simulink library "PB_Library_Master_Working"  (R2021a)
settings: Solver=VariableStepAuto  StartTime=0.0  StopTime=10.0  RelTol=1e-3
undefined symbols (not defined in the file): A_M, B_M, component_degradation_input, E0_M, f_sw, f_sw_M_aDF, flux_m_aDF, Fsw_M_aDF, insert, K_M, L_M_aDF, L_M_adf, P_Fe_Nom_aDF, Q_M, Q_rr, r_c, r_D, R_M, R_s_aDF, resistance_aDF, S_nom_aDF, SOC_Init_M, TFall_M_aDF, TRise_M_aDF, Trr_M_aDF, u_ce0, u_D0
libraries: $bdroot x76, Lib_Dyn_StateSpace_EMTAT x6, Lib_PF_BusLoadDC_TMATS x3, PB_Library_Master x3, simulink x3, TemperatureBlock x1
(part 2 of 5)

== system PB_Library_Master_Working/Boost Converter ==
  Vin : Inport
  IgIn : Inport  Port=2
  x : Inport  Port=3
  d : Inport  Port=4
  dt : Inport  Port=5
  Iout : Inport  Port=6
  Temp (Rankine) : Inport  Port=7  Unit=degC
  Bus : Lib_PF_BusLoadDC_TMATS/LoadBus DC  P_M=-Pdis_M  BlkNm_M=double(gcb)
  Bus Creator : BusCreator  Inputs=11
  DC - DC Converter : Subsystem
      mask Display:
      | fprintf('Boost')
      | 
      | port_label('input',1,'VA')
      | port_label('input',2,'IAg')
      | port_label('input',3,'x')
      | port_label('input',4,'d')
      | port_label('input',5,'dt')
      | port_label('input',6,'Iout')
      | port_label('input',7,'Ploss')
      | 
      | 
      | port_label('output',1,'VB')
      | port_label('output',2,'x_dot')
      | port_label('output',3,'x_new')
      | port_label('output',4,'PElec')
      | port_label('output',5,'IA')
      | port_label('output',6,'switchDyn')
  Display : Display
  "Power Loss " : Subsystem
  Product1 : Product
  Product3 : Product
  Rankine to Celsius : PB_Library_Master/Rankine to Celsius  SystemSampleTime=-1  VariantActivationTime=update diagram  Latency=0  AutoFrameSizeCalculation=off
  "TempConv " : Subsystem  Commented=on
      mask DialogControl DescTextVar Prompt: Temperature Unit Converter
  Terminator3 : Terminator
  Vout : Outport  VectorParamsAs1DForOutWhenUnconnected=off
  xdot : Outport  Port=2  VectorParamsAs1DForOutWhenUnconnected=off
  x_new : Outport  Port=3  VectorParamsAs1DForOutWhenUnconnected=off
  P_err : Outport  Port=4  VectorParamsAs1DForOutWhenUnconnected=off
  Outputs : Outport  Port=5  VectorParamsAs1DForOutWhenUnconnected=off
  Iin : Outport  Port=6  VectorParamsAs1DForOutWhenUnconnected=off
  Heat (W) : Outport  Port=7  VectorParamsAs1DForOutWhenUnconnected=off
  wires:
  DC - DC Converter/4(PElec) -> Bus/2
  Temp (Rankine)/1 -> Rankine to Celsius/1, Display/1  "TempIn"
  Rankine to Celsius/1 -> DC - DC Converter/8("T_Ambient "), "Power Loss "/5("T_Ambient ")
  DC - DC Converter/6(switchDyn) -> Bus Creator/1  "switchDyn"
  dt/1 -> DC - DC Converter/5(dt)
  DC - DC Converter/3(x_new) -> x_new/1, Bus Creator/10  "x"
  "Power Loss "/1(" P loss") -> Heat (W)/1, Bus Creator/3, DC - DC Converter/7(P loss)  "P loss"
  d/1 -> DC - DC Converter/4(d), "Power Loss "/3(d)
  x/1 -> DC - DC Converter/3(x)
  IgIn/1 -> DC - DC Converter/2(IAg)
  DC - DC Converter/5(IA) -> Iin/1, Bus Creator/2, Product3/2  "Iin"
  DC - DC Converter/2(x_dot) -> xdot/1, Bus Creator/11  "x_dot"
  Iout/1 -> Bus Creator/5, Product1/1, Bus/3, "Power Loss "/2(Iout), DC - DC Converter/6(Iout)  "Iout"
  Bus/1 -> Vout/1, "Power Loss "/4(Vout)
  Product1/1 -> Bus Creator/7  "Pout"
  Product3/1 -> Bus Creator/6  "Pin"
  Vin/1 -> Bus Creator/4, Product3/1, "Power Loss "/1(Vin), DC - DC Converter/1(NodeA)  "Vin"
  DC - DC Converter/1(NodeB) -> Bus/1, Product1/2
  Bus/3 -> Terminator3/1
  Bus/2 -> P_err/1
  Bus Creator/1 -> Outputs/1
  "Power Loss "/3(RippleV) -> Bus Creator/9  "Ripple V"
  "Power Loss "/2(RippleI) -> Bus Creator/8  "Ripple I"

== system PB_Library_Master_Working/Boost Converter Analytic ==
  Vin : Inport
  x : Inport  Port=2
  d : Inport  Port=3
  dt : Inport  Port=4
  Iout : Inport  Port=5
  Temp (Rankine) : Inport  Port=6  Unit=degC
  FaultToggle : Inport  Port=7
  Bus Creator : BusCreator  Inputs=11
  Catastrophic Fault Block{,1..6} (7 alike) : $bdroot/Catastrophic Fault Block  SystemSampleTime=-1  VariantActivationTime=update diagram  Latency=0  AutoFrameSizeCalculation=off
  DC - DC Converter : Subsystem
  Display : Display
  Divide : Product  Inputs=*/
  Divide1 : Product  Inputs=*/
  "Power Loss " : Subsystem
  Product1 : Product
  Product3 : Product
  Rankine to Celsius : PB_Library_Master/Rankine to Celsius  SystemSampleTime=-1  VariantActivationTime=update diagram  Latency=0  AutoFrameSizeCalculation=off
  Switch : Switch  Criteria=u2 > Threshold
  "TempConv " : Subsystem  Commented=on
      mask DialogControl DescTextVar Prompt: Temperature Unit Converter
  Voltage Catastrophic Fault Block : $bdroot/Voltage Catastrophic Fault Block  SystemSampleTime=-1  VariantActivationTime=update diagram  Latency=0  AutoFrameSizeCalculation=off
  Vout : Outport  VectorParamsAs1DForOutWhenUnconnected=off
  xdot : Outport  Port=2  VectorParamsAs1DForOutWhenUnconnected=off
  x_new : Outport  Port=3  VectorParamsAs1DForOutWhenUnconnected=off
  Outputs : Outport  Port=4  VectorParamsAs1DForOutWhenUnconnected=off
  Iin : Outport  Port=5  VectorParamsAs1DForOutWhenUnconnected=off
  Heat (W) : Outport  Port=6  VectorParamsAs1DForOutWhenUnconnected=off
  Eff : Outport  Port=7  VectorParamsAs1DForOutWhenUnconnected=off
  wires:
  Temp (Rankine)/1 -> Rankine to Celsius/1, Display/1  "TempIn"
  Rankine to Celsius/1 -> DC - DC Converter/7("T_Ambient "), "Power Loss "/5("T_Ambient ")
  DC - DC Converter/5(switchDyn) -> Bus Creator/1  "switchDyn"
  dt/1 -> DC - DC Converter/4(dt)
  DC - DC Converter/3(x_new) -> Catastrophic Fault Block2/2, Bus Creator/10  "x"
  "Power Loss "/1(" P loss") -> Bus Creator/3, Catastrophic Fault Block5/2, DC - DC Converter/6(P loss)  "P loss"
  d/1 -> DC - DC Converter/3(d), "Power Loss "/3(d)
  x/1 -> DC - DC Converter/2(x)
  DC - DC Converter/4(I_Demanded) -> Product3/2, Catastrophic Fault Block3/2, Bus Creator/2  "Iin"
  DC - DC Converter/2(x_dot) -> Catastrophic Fault Block1/2, Bus Creator/11  "x_dot"
  Iout/1 -> "Power Loss "/2(Iout), DC - DC Converter/5(I_Demand), Switch/2, Bus Creator/5, Product1/1  "Iout"
  DC - DC Converter/1(VOut) -> Catastrophic Fault Block/2, "Power Loss "/4(Vout), Product1/2
  Product1/1 -> Divide1/1, Bus Creator/7, Divide/2  "Pout"
  Product3/1 -> Divide1/2, Bus Creator/6, Divide/1  "Pin"
  "Power Loss "/3(RippleV) -> Bus Creator/9  "Ripple V"
  "Power Loss "/2(RippleI) -> Bus Creator/8  "Ripple I"
  Catastrophic Fault Block/1 -> Vout/1
  [FT] -> Catastrophic Fault Block/1
  [FT] -> Catastrophic Fault Block1/1
  Catastrophic Fault Block1/1 -> xdot/1
  Voltage Catastrophic Fault Block/2 -> DC - DC Converter/1(VIn), "Power Loss "/1(Vin), Product3/1, Bus Creator/4  "Vin"
  Vin/1 -> Voltage Catastrophic Fault Block/2  "Vin"
  FaultToggle/1 -> Voltage Catastrophic Fault Block/1
  Voltage Catastrophic Fault Block/1 -> [FT]
  [FT] -> Catastrophic Fault Block2/1
  Catastrophic Fault Block2/1 -> x_new/1
  [FT] -> Catastrophic Fault Block3/1
  Catastrophic Fault Block3/1 -> Iin/1
  [FT] -> Catastrophic Fault Block4/1
  Bus Creator/1 -> Catastrophic Fault Block4/2
  Catastrophic Fault Block4/1 -> Outputs/1
  [FT] -> Catastrophic Fault Block5/1
  Catastrophic Fault Block5/1 -> Heat (W)/1
  Catastrophic Fault Block6/1 -> Eff/1
  [FT] -> Catastrophic Fault Block6/1
  Switch/1 -> Catastrophic Fault Block6/2
  Divide1/1 -> Switch/1
  Divide/1 -> Switch/3

== system PB_Library_Master_Working/Buck Converter ==
  Vin : Inport
  IgIn : Inport  Port=2
  x : Inport  Port=3
  d : Inport  Port=4
  dt : Inport  Port=5
  Iout : Inport  Port=6
  T_Ambient : Inport  Port=7  Unit=degC
  Bus : Lib_PF_BusLoadDC_TMATS/LoadBus DC  P_M=-Pdis_M  BlkNm_M=double(gcb)
  Bus Creator : BusCreator  Inputs=11
  DC - DC Converter : Subsystem
      mask Display:
      | fprintf('Buck')
      | 
      | port_label('input',1,'VA')
      | port_label('input',2,'IAg')
      | port_label('input',3,'x')
      | port_label('input',4,'d')
      | port_label('input',5,'dt')
      | port_label('input',6,'Iout')
      | port_label('input',7,'Ploss')
      | 
      | 
      | port_label('output',1,'VB')
      | port_label('output',2,'x_dot')
      | port_label('output',3,'x_new')
      | port_label('output',4,'PElec')
      | port_label('output',5,'IA')
      | port_label('output',6,'switchDyn')
  "Power Loss " : Subsystem
  Product1 : Product
  Product3 : Product
  Rankine to Celsius : $bdroot/Rankine to Celsius  SystemSampleTime=-1  VariantActivationTime=update diagram  Latency=0  AutoFrameSizeCalculation=off
  "TempConv " : Subsystem  Commented=on
      mask DialogControl DescTextVar Prompt: Temperature Unit Converter
  Terminator3 : Terminator
  Vout : Outport  VectorParamsAs1DForOutWhenUnconnected=off
  xdot : Outport  Port=2  VectorParamsAs1DForOutWhenUnconnected=off
  x_new : Outport  Port=3  VectorParamsAs1DForOutWhenUnconnected=off
  P_err : Outport  Port=4  VectorParamsAs1DForOutWhenUnconnected=off
  Outputs : Outport  Port=5  VectorParamsAs1DForOutWhenUnconnected=off
  Iin : Outport  Port=6  VectorParamsAs1DForOutWhenUnconnected=off
  Heat : Outport  Port=7  VectorParamsAs1DForOutWhenUnconnected=off
  wires:
  Rankine to Celsius/1 -> DC - DC Converter/8("T_Ambient "), "Power Loss "/5("T_Ambient ")
  T_Ambient/1 -> Rankine to Celsius/1
  DC - DC Converter/6(switchDyn) -> Bus Creator/1  "switchDyn"
  dt/1 -> DC - DC Converter/5(dt)
  DC - DC Converter/3(x_new) -> x_new/1, Bus Creator/10  "x"
  "Power Loss "/1(" P loss") -> Bus Creator/3, Heat/1, DC - DC Converter/7(P loss)  "P loss"
  d/1 -> "Power Loss "/3(d), DC - DC Converter/4(d)
  x/1 -> DC - DC Converter/3(x)
  DC - DC Converter/5(IA) -> Iin/1, Bus Creator/2, Product3/2  "Iin"
  DC - DC Converter/4(PElec) -> Bus/2
  DC - DC Converter/2(x_dot) -> xdot/1, Bus Creator/11  "x_dot"
  Iout/1 -> Bus/3, Bus Creator/5, Product1/1, "Power Loss "/2(Iout), DC - DC Converter/6(Iout)  "Iout"
  Bus/1 -> "Power Loss "/4(Vout), Vout/1
  Product1/1 -> Bus Creator/7  "Pout"
  Product3/1 -> Bus Creator/6  "Pin"
  DC - DC Converter/1(NodeB) -> Bus/1, Product1/2
  Bus/3 -> Terminator3/1
  Bus/2 -> P_err/1
  Bus Creator/1 -> Outputs/1
  "Power Loss "/3(RippleV) -> Bus Creator/9  "Ripple V"
  "Power Loss "/2(RippleI) -> Bus Creator/8  "Ripple I"
  IgIn/1 -> DC - DC Converter/2(IAg)
  Vin/1 -> Bus Creator/4, Product3/1, "Power Loss "/1(Vin), DC - DC Converter/1(NodeA)  "Vin"

== system PB_Library_Master_Working/Buck Converter Analytic ==
  Vin : Inport
  x : Inport  Port=2
  d : Inport  Port=3
  dt : Inport  Port=4
  I_Demand : Inport  Port=5
  T_Ambient : Inport  Port=6  Unit=degC
  FaultToggle : Inport  Port=7  Unit=degC
  Bus Creator : BusCreator  Inputs=11
  Catastrophic Fault Block{1..7} (7 alike) : $bdroot/Catastrophic Fault Block  SystemSampleTime=-1  VariantActivationTime=update diagram  Latency=0  AutoFrameSizeCalculation=off
  DC - DC Converter : Subsystem
  Divide : Product  Inputs=*/
  Divide1 : Product  Inputs=*/
  "Power Loss " : Subsystem
  Product1 : Product
  Product3 : Product
  Rankine to Celsius : PB_Library_Master/Rankine to Celsius  SystemSampleTime=-1  VariantActivationTime=update diagram  Latency=0  AutoFrameSizeCalculation=off
  Switch : Switch  Criteria=u2 > Threshold
  "TempConv " : Subsystem  Commented=on
      mask DialogControl DescTextVar Prompt: Temperature Unit Converter
  Vout : Outport  VectorParamsAs1DForOutWhenUnconnected=off
  xdot : Outport  Port=2  VectorParamsAs1DForOutWhenUnconnected=off
  x_new : Outport  Port=3  VectorParamsAs1DForOutWhenUnconnected=off
  Outputs : Outport  Port=4  VectorParamsAs1DForOutWhenUnconnected=off
  I_Demanded : Outport  Port=5  VectorParamsAs1DForOutWhenUnconnected=off
  Heat : Outport  Port=6  VectorParamsAs1DForOutWhenUnconnected=off
  Eff : Outport  Port=7  VectorParamsAs1DForOutWhenUnconnected=off
  wires:
  Vin/1 -> DC - DC Converter/1(VIn), "Power Loss "/1(Vin), Product3/1, Bus Creator/4  "Vin"
  "Power Loss "/2(RippleI) -> Bus Creator/8  "Ripple I"
  "Power Loss "/3(RippleV) -> Bus Creator/9  "Ripple V"
  DC - DC Converter/1(Vout) -> Catastrophic Fault Block4/2, "Power Loss "/4(Vout), Product1/2
  DC - DC Converter/2(x_dot) -> Catastrophic Fault Block1/2, Bus Creator/11  "x_dot"
  DC - DC Converter/4(I_Demanded) -> Catastrophic Fault Block3/2, Bus Creator/2, Product3/2  "Iin"
  x/1 -> DC - DC Converter/2(x)
  d/1 -> "Power Loss "/3(d), DC - DC Converter/3(d)
  "Power Loss "/1(" P loss") -> DC - DC Converter/6(P loss), Bus Creator/3, Catastrophic Fault Block6/2  "P loss"
  DC - DC Converter/3(x_new) -> Bus Creator/10, Catastrophic Fault Block2/2  "x"
  dt/1 -> DC - DC Converter/4(dt)
  DC - DC Converter/5(switchDyn) -> Bus Creator/1  "switchDyn"
  T_Ambient/1 -> Rankine to Celsius/1
  Rankine to Celsius/1 -> "Power Loss "/5("T_Ambient "), DC - DC Converter/7("T_Ambient ")
  [FT] -> Catastrophic Fault Block4/1
  Catastrophic Fault Block4/1 -> Vout/1
  [FT] -> Catastrophic Fault Block1/1
  Catastrophic Fault Block1/1 -> xdot/1
  [FT] -> Catastrophic Fault Block2/1
  Catastrophic Fault Block2/1 -> x_new/1
  [FT] -> Catastrophic Fault Block3/1
  Catastrophic Fault Block3/1 -> I_Demanded/1
  [FT] -> Catastrophic Fault Block5/1
  Bus Creator/1 -> Catastrophic Fault Block5/2
  Catastrophic Fault Block5/1 -> Outputs/1
  [FT] -> Catastrophic Fault Block6/1
  Catastrophic Fault Block6/1 -> Heat/1
  FaultToggle/1 -> [FT]
  Catastrophic Fault Block7/1 -> Eff/1
  [FT] -> Catastrophic Fault Block7/1
  Product3/1 -> Divide1/2, Divide/1, Bus Creator/6  "Pin"
  Product1/1 -> Divide1/1, Divide/2, Bus Creator/7  "Pout"
  Divide1/1 -> Switch/1
  Divide/1 -> Switch/3
  I_Demand/1 -> "Power Loss "/2(Iout), Product1/1, Switch/2, Bus Creator/5, DC - DC Converter/5(I_Demand)  "Iout"
  Switch/1 -> Catastrophic Fault Block7/2

== system PB_Library_Master_Working/Cable_iDesign ==
  note: UPDATE RESISTANCE BASED ON AMBIENT TEMPERATURE CHANGE
  note: GENERAL ELECTRICAL CALCULATIONS
  note: ------------------------------------------------
      | Created by Nathan Butler
      | NASA Glenn Research Center
      | MATLAB R2020b
      | Spring 2021
      | ------------------------------------------------
  Idemand : Inport
  Vin : Inport  Port=2
  Temp : Inport  Port=3
  FaultToggle : Inport  Port=4
  Add : Sum
  Catastrophic Fault Block : $bdroot/Catastrophic Fault Block  SystemSampleTime=-1  VariantActivationTime=update diagram  Latency=0  AutoFrameSizeCalculation=off
  Catastrophic Fault Block1 : $bdroot/Catastrophic Fault Block  SystemSampleTime=-1  VariantActivationTime=update diagram  Latency=0  AutoFrameSizeCalculation=off
  Catastrophic Fault Block2 : $bdroot/Catastrophic Fault Block  SystemSampleTime=-1  VariantActivationTime=update diagram  Latency=0  AutoFrameSizeCalculation=off
  Constant : Constant  Value=alpha
  Constant1 : Constant
  Constant3 : Constant  Value=R_init
  I_dmd*Vdrop : Product
  Product : Product
  Product1 : Product
  Product3 : Product
  Rankine to Celsius : $bdroot/Rankine to Celsius  SystemSampleTime=-1  VariantActivationTime=update diagram  Latency=0  AutoFrameSizeCalculation=off
  Ref Temp (C) : Constant  Value=20
  Subtract1 : Sum  Inputs=+-
  Vin-Vdrop : Sum  Inputs=+-
  Voltage Catastrophic Fault Block : $bdroot/Voltage Catastrophic Fault Block  SystemSampleTime=-1  VariantActivationTime=update diagram  Latency=0  AutoFrameSizeCalculation=off
  Idemanded : Outport  VectorParamsAs1DForOutWhenUnconnected=off
  Vout : Outport  Port=2  VectorParamsAs1DForOutWhenUnconnected=off
  Heat : Outport  Port=3  VectorParamsAs1DForOutWhenUnconnected=off
  wires:
  Subtract1/1 -> Product/2  "delta_T"
  Constant/1 -> Product/1
  Product/1 -> Add/2
  Constant1/1 -> Add/1
  Add/1 -> Product1/1  "1+alpha(deltaT)"
  Product1/1 -> [R]  "R2"
  Constant3/1 -> Product1/2
  Ref Temp (C)/1 -> Subtract1/2
  Vin-Vdrop/1 -> Catastrophic Fault Block1/2
  Idemand/1 -> Product3/1, Catastrophic Fault Block/2, I_dmd*Vdrop/2
  [R] -> Product3/2
  Product3/1 -> I_dmd*Vdrop/1, Vin-Vdrop/2  "VDrop"
  Temp/1 -> Rankine to Celsius/1
  Rankine to Celsius/1 -> Subtract1/1
  Catastrophic Fault Block/1 -> Idemanded/1
  [FT] -> Catastrophic Fault Block/1
  [FT] -> Catastrophic Fault Block1/1
  [FT] -> Catastrophic Fault Block2/1
  I_dmd*Vdrop/1 -> Catastrophic Fault Block2/2
  Catastrophic Fault Block2/1 -> Heat/1
  Catastrophic Fault Block1/1 -> Vout/1
  Vin/1 -> Voltage Catastrophic Fault Block/2
  Voltage Catastrophic Fault Block/2 -> Vin-Vdrop/1
  Voltage Catastrophic Fault Block/1 -> [FT]
  FaultToggle/1 -> Voltage Catastrophic Fault Block/1

== system PB_Library_Master_Working/Catastrophic Fault Block ==
  Fault Toggle : Inport
  Inport Value : Inport  Port=2
  Display{,1..3} (4 alike) : Display
  OR1 : Logic  Operator=OR  IconShape=distinctive  AllPortsSameDT=off  OutDataTypeStr=boolean
  Relational Operator : RelationalOperator  Operator=isInf  OutDataTypeStr=boolean  RndMeth=Simplest
  Relational Operator3 : RelationalOperator  Operator=isNaN  OutDataTypeStr=boolean  RndMeth=Simplest
  Switch1 : Switch  Criteria=u2 > Threshold
  Switch2 : Switch  Criteria=u2 > Threshold
  Zero1 : Constant  Value=0
  Zero2 : Constant  Value=0
  Outport Value : Outport
  wires:
  Fault Toggle/1 -> Switch2/2
  Zero2/1 -> Switch1/1
  Zero1/1 -> Switch2/1
  Inport Value/1 -> Switch2/3
  OR1/1 -> Display2/1, Switch1/2
  Relational Operator3/1 -> OR1/2
  Relational Operator/1 -> OR1/1
  Switch1/1 -> Display1/1, Outport Value/1
  Switch2/1 -> Display3/1, Display/1, Switch1/3, Relational Operator3/1, Relational Operator/1

== system PB_Library_Master_Working/Degradation Input Block ==
  Degradation Input Value : Constant  Value=component_degradation_input
  Disp Degradation Input : Display
  Disp Original Degradation Factor : Display
  Exp : Math  Operator=10^u  SaturateOnIntegerOverflow=on
  Reciprocal : Product  Inputs=/
  Degradation Factor : Outport
  Degradation Input : Outport  Port=2
  wires:
  Degradation Input Value/1 -> Exp/1, Degradation Input/1, Disp Degradation Input/1
  Exp/1 -> Reciprocal/1
  Reciprocal/1 -> Disp Original Degradation Factor/1, Degradation Factor/1

== system PB_Library_Master_Working/Degradation Parameter Multiplier ==
  Parameter Adjustment : Inport
  Display{,1..4} (5 alike) : Display
  Exp1 : Math  Operator=10^u  SaturateOnIntegerOverflow=on
  Product3 : Product
  Product4 : Product
  Adjusted Degradation Factor : Outport
  wires:
  Parameter Adjustment/1 -> Product4/2
  Product4/1 -> Display3/1, Exp1/1
  [component_DI] -> Display4/1, Product4/1
  Product3/1 -> Display/1, Adjusted Degradation Factor/1
  Exp1/1 -> Display2/1, Product3/1
  [component_DF] -> Display1/1, Product3/2

== system PB_Library_Master_Working/Electrothermal_Battery_Model ==
  note: Electrical Model
  note: Bus Library Block
  it_base : Inport
  IgIn : Inport  Port=2
  Iout : Inport  Port=3
  Temp (Ra) : Inport  Port=4  Unit=degC
  Battery Core (w/ Q) : Subsystem
  Bus : Lib_PF_BusLoadDC_TMATS/LoadBus DC  P_M=0  BlkNm_M=double(gcb)
  Bus Creator : BusCreator  Inputs=7
  Product1 : Product
  Rankine to Celsius : $bdroot/Rankine to Celsius  SystemSampleTime=-1  VariantActivationTime=update diagram  Latency=0  AutoFrameSizeCalculation=off
  "TempConv " : Subsystem  Commented=on
      mask DialogControl DescTextVar Prompt: Temperature Unit Converter
  Terminator3 : Terminator
  it_Dot = f(i) : Subsystem
  Vout : Outport  VectorParamsAs1DForOutWhenUnconnected=off
  P_err : Outport  Port=2  VectorParamsAs1DForOutWhenUnconnected=off
  Outputs : Outport  Port=3  VectorParamsAs1DForOutWhenUnconnected=off
  it_Dot : Outport  Port=4  VectorParamsAs1DForOutWhenUnconnected=off
  Heat : Outport  Port=5  VectorParamsAs1DForOutWhenUnconnected=off
  wires:
  Rankine to Celsius/1 -> Battery Core (w/ Q)/3(Tavg)
  Battery Core (w/ Q)/3(it) -> Bus Creator/6  "it"
  Battery Core (w/ Q)/2(SOC) -> Bus Creator/4  "SOC"
  it_base/1 -> Battery Core (w/ Q)/1(it_base)
  Battery Core (w/ Q)/1(Vout) -> Bus/1, Bus Creator/1, Product1/1  "Vout"
  Product1/1 -> Bus/2, Bus Creator/3  "Pout"
  [Iout] -> Bus/3
  Bus/2 -> P_err/1
  Bus/3 -> Terminator3/1
  Iout/1 -> it_Dot = f(i)/1(i), [Iout]
  Bus/1 -> Vout/1
  it_Dot = f(i)/1(it_Dot) -> Bus Creator/5, it_Dot/1  "it_Dot"
  IgIn/1 -> Battery Core (w/ Q)/2(IgIn), Product1/2, Bus Creator/2  "Iout"
  Bus Creator/1 -> Outputs/1
  Battery Core (w/ Q)/4(Heat_Generated) -> Heat/1, Bus Creator/7  "Heat_Generated"
  Temp (Ra)/1 -> Rankine to Celsius/1

== system PB_Library_Master_Working/Electrothermal_Battery_Model_Analytic ==
  note: Electrical Model
  it_base : Inport
  I_Demand : Inport  Port=2
  Temp (Ra) : Inport  Port=3  Unit=degC
  FaultToggle : Inport  Port=4  Unit=degC
  Battery Core (w/ Q) : Subsystem
  Bus Creator : BusCreator  Inputs=7
  Catastrophic Fault Block{,1..5} (6 alike) : $bdroot/Catastrophic Fault Block  SystemSampleTime=-1  VariantActivationTime=update diagram  Latency=0  AutoFrameSizeCalculation=off
  Degradation Input Block : $bdroot/Degradation Input Block  SystemSampleTime=-1  VariantActivationTime=update diagram  Latency=0  AutoFrameSizeCalculation=off
  Product1 : Product
  Rankine to Celsius : $bdroot/Rankine to Celsius  SystemSampleTime=-1  VariantActivationTime=update diagram  Latency=0  AutoFrameSizeCalculation=off
  it_Dot = f(i) : Subsystem
  Vout : Outport  VectorParamsAs1DForOutWhenUnconnected=off
  Outputs : Outport  Port=2  VectorParamsAs1DForOutWhenUnconnected=off
  it_Dot : Outport  Port=3  VectorParamsAs1DForOutWhenUnconnected=off
  Heat : Outport  Port=4  VectorParamsAs1DForOutWhenUnconnected=off
  SOC : Outport  Port=5  VectorParamsAs1DForOutWhenUnconnected=off
  it : Outport  Port=6  VectorParamsAs1DForOutWhenUnconnected=off
  wires:
  Rankine to Celsius/1 -> Battery Core (w/ Q)/3(Tavg)
  Battery Core (w/ Q)/3(it) -> Bus Creator/6, Catastrophic Fault Block5/2  "it"
  Battery Core (w/ Q)/2(SOC) -> Catastrophic Fault Block4/2, Bus Creator/4  "SOC"
  it_base/1 -> Battery Core (w/ Q)/1(it_base)
  Battery Core (w/ Q)/1(Vout) -> Catastrophic Fault Block/2, Bus Creator/1, Product1/1  "Vout"
  Product1/1 -> Bus Creator/3  "Pout"
  it_Dot = f(i)/1(it_Dot) -> Catastrophic Fault Block2/2, Bus Creator/5  "it_Dot"
  I_Demand/1 -> it_Dot = f(i)/1(i), Battery Core (w/ Q)/2(I_Demand), Bus Creator/2, Product1/2  "Iout"
  Battery Core (w/ Q)/4(Heat_Generated) -> Bus Creator/7, Catastrophic Fault Block3/2  "Heat_Generated"
  Temp (Ra)/1 -> Rankine to Celsius/1
  Catastrophic Fault Block/1 -> Vout/1
  FaultToggle/1 -> [FT]
  [FT] -> Catastrophic Fault Block/1
  [FT] -> Catastrophic Fault Block1/1
  Bus Creator/1 -> Catastrophic Fault Block1/2
  Catastrophic Fault Block1/1 -> Outputs/1
  [FT] -> Catastrophic Fault Block2/1
  Catastrophic Fault Block2/1 -> it_Dot/1
  [FT] -> Catastrophic Fault Block3/1
  Catastrophic Fault Block3/1 -> Heat/1
  Catastrophic Fault Block4/1 -> SOC/1
  [FT] -> Catastrophic Fault Block4/1
  Catastrophic Fault Block5/1 -> it/1
  [FT] -> Catastrophic Fault Block5/1
  Degradation Input Block/1 -> [A]
  Degradation Input Block/2 -> [A]

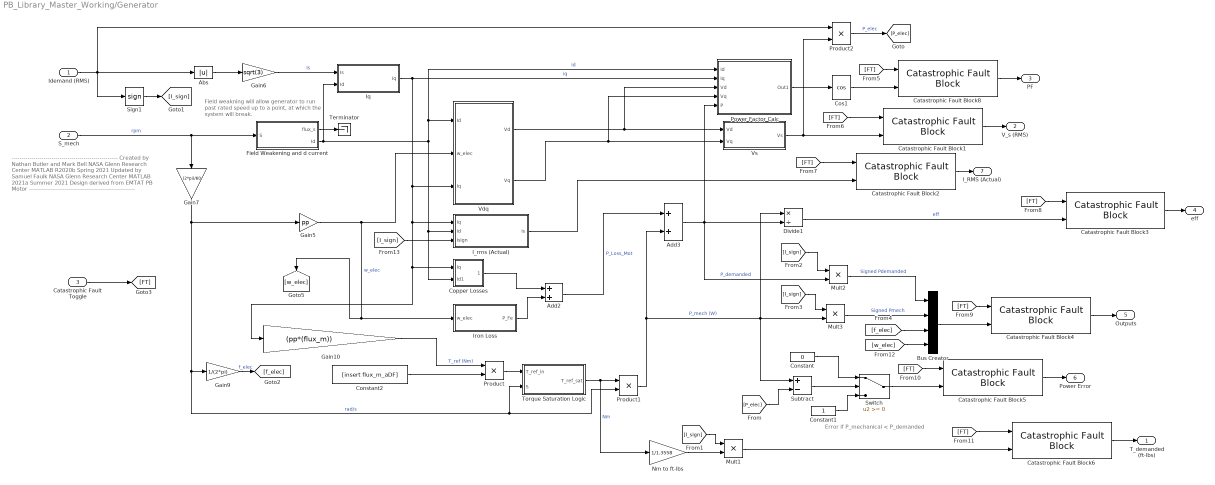
== system PB_Library_Master_Working/Generator ==
  note: Field weakning will allow generator to run past rated speed up to a point, at which the system will break.
  note: Error if P_mechanical < P_demanded
  note: -----------------------------------------------------
      | Created by Nathan Butler and Mark Bell
      | NASA Glenn Research Center
      | MATLAB R2020b
      | Spring 2021
      |
      | Updated by Samuel Faulk
      | NASA Glenn Research Center
      | MATLAB 2021a
      | Summer 2021
      |
      | Design derived from EMTAT PB Motor
      | -----------------------------------------------------
  Idemand (RMS) : Inport
  S_mech : Inport  Port=2
  Catastrophic Fault Toggle : Inport  Port=3
  Abs : Abs
  Add2 : Sum
  Add3 : Sum
  Bus Creator : BusCreator  Inputs=4
  Catastrophic Fault Block{1..6,8} (7 alike) : $bdroot/Catastrophic Fault Block  SystemSampleTime=-1  VariantActivationTime=update diagram  Latency=0  AutoFrameSizeCalculation=off
  Constant : Constant  Value=0
  Constant1 : Constant
  Constant2 : Constant  Value=[insert flux_m_aDF]
  Copper Losses : Subsystem
  Cos1 : Trigonometry  Operator=cos
  Divide1 : Product  Inputs=*/
  "Field Weakening and d current " : Subsystem
  Gain10 : Gain  Gain=(pp*(flux_m))
  Gain5 : Gain  Gain=pp
  Gain6 : Gain  Gain=sqrt(3)
  Gain7 : Gain  Gain=(2*pi)/60
  Gain9 : Gain  Gain=1/(2*pi)
  I_rms (Actual) : Subsystem
  Iq : Subsystem
  Iron Loss : Subsystem
  Mult1 : Product  Inputs=**
  Mult2 : Product  Inputs=**
  Mult3 : Product  Inputs=**
  Nm to ft-lbs : Gain  Gain=1/1.3558
  Power Factor Calc : Subsystem
  Product : Product
  Product1 : Product
  Product2 : Product
  Sign1 : Signum
  Subtract : Sum  Inputs=+-
  Switch : Switch
  Terminator : Terminator
  Torque Saturation Logic : Subsystem
  Vdq : Subsystem
  Vs : Subsystem
  T_demanded (ft-lbs) : Outport
  V_s (RMS) : Outport  Port=2
  PF : Outport  Port=3
  eff : Outport  Port=4
  Outputs : Outport  Port=5
  Power Error : Outport  Port=6
  I_RMS (Actual) : Outport  Port=7
  wires:
  Add3/1 -> Power Factor Calc/5(P), Divide1/2, Mult2/2  "P_demanded"
  [w_elec] -> Bus Creator/4
  [f_elec] -> Bus Creator/3
  Gain9/1 -> [f_elec]  "f_elec"
  Mult3/1 -> Bus Creator/2  "Signed Pmech"
  Mult2/1 -> Bus Creator/1  "Signed Pdemanded"
  [I_sign] -> Mult3/1
  [I_sign] -> Mult2/1
  [I_sign] -> Mult1/1
  Sign1/1 -> [I_sign]
  Idemand (RMS)/1 -> Abs/1, Sign1/1, Product2/1
  Torque Saturation Logic/1(T_ref_sat) -> Nm to ft-lbs/1, Product1/1  "Nm"
  "Field Weakening and d current "/1(flux_s) -> Terminator/1
  Gain6/1 -> Iq/1(Is)  "Is"
  Product1/1 -> Mult3/2, Divide1/1, Subtract/1, Add3/2  "P_mech (W)"
  Iq/1(Iq) -> Power Factor Calc/2(Iq), Gain10/1, Copper Losses/1(Iq), I_rms (Actual)/1(iq), Vdq/3(Iq)  "iq"
  S_mech/1 -> "Field Weakening and d current "/1(S), Gain7/1  "rpm"
  "Field Weakening and d current "/2(Id) -> Copper Losses/2(Id1), I_rms (Actual)/2(id), Power Factor Calc/1(Id), Vdq/1(Id), Iq/2(Id)  "id"
  Gain5/1 -> Iron Loss/1(w_elec), [w_elec], Vdq/2(w_elec)  "w_elec"
  Vdq/1(Vd) -> Vs/1(Vd), Power Factor Calc/3(Vd)
  Vdq/2(Vq) -> Vs/2(Vq), Power Factor Calc/4(Vq)
  Vs/1(Vs) -> Catastrophic Fault Block1/2, Product2/2
  Copper Losses/1(P_Cu) -> Add2/1
  Iron Loss/1(P_Fe) -> Add2/2
  Add2/1 -> Add3/1  "P_Loss_Mot"
  Power Factor Calc/1(Out1) -> Cos1/1
  Subtract/1 -> Switch/2
  Constant/1 -> Switch/1
  Constant1/1 -> Switch/3
  Product2/1 -> [P_elec]  "P_elec"
  [P_elec] -> Subtract/2
  Nm to ft-lbs/1 -> Mult1/2
  Gain7/1 -> Gain5/1, Gain9/1, Torque Saturation Logic/2(S), Product1/2  "rad/s"
  Abs/1 -> Gain6/1
  [FT] -> Catastrophic Fault Block8/1
  Cos1/1 -> Catastrophic Fault Block8/2
  Catastrophic Fault Block8/1 -> PF/1
  [FT] -> Catastrophic Fault Block1/1
  Catastrophic Fault Block1/1 -> V_s (RMS)/1
  [FT] -> Catastrophic Fault Block2/1
  Catastrophic Fault Block2/1 -> I_RMS (Actual)/1
  I_rms (Actual)/1(Is) -> Catastrophic Fault Block2/2
  [FT] -> Catastrophic Fault Block3/1
  Divide1/1 -> Catastrophic Fault Block3/2  "eff"
  Catastrophic Fault Block3/1 -> eff/1
  [FT] -> Catastrophic Fault Block4/1
  Bus Creator/1 -> Catastrophic Fault Block4/2
  Catastrophic Fault Block4/1 -> Outputs/1
  [FT] -> Catastrophic Fault Block5/1
  Switch/1 -> Catastrophic Fault Block5/2
  Catastrophic Fault Block5/1 -> Power Error/1
  [FT] -> Catastrophic Fault Block6/1
  Mult1/1 -> Catastrophic Fault Block6/2
  Catastrophic Fault Block6/1 -> T_demanded (ft-lbs)/1
  [I_sign] -> I_rms (Actual)/3(Isign)
  Catastrophic Fault Toggle/1 -> [FT]
  Product/1 -> Torque Saturation Logic/1(T_ref_in)
  Gain10/1 -> Product/1  "T_ref (Nm)"
  Constant2/1 -> Product/2

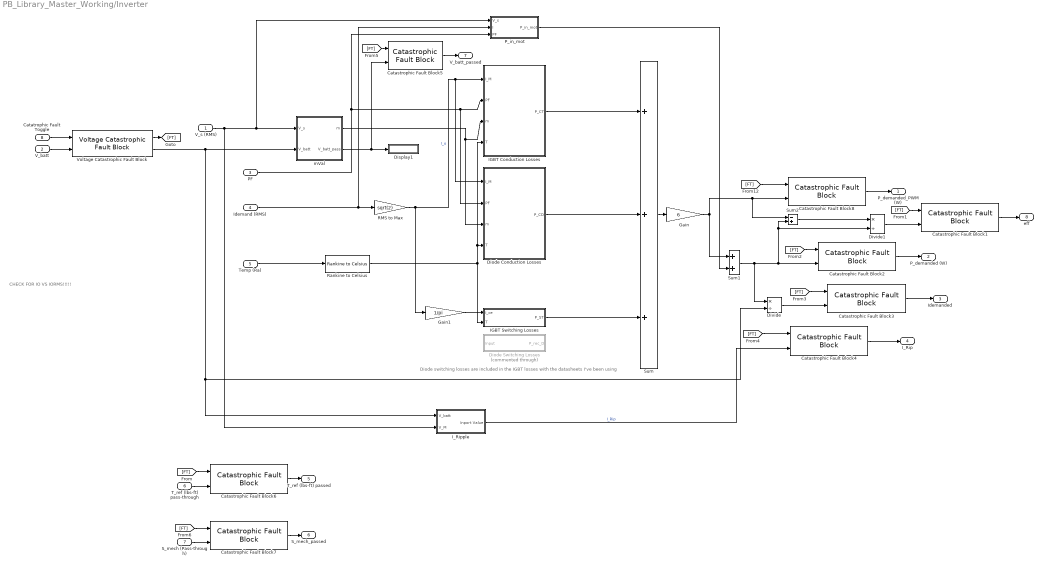
== system PB_Library_Master_Working/Inverter ==
  note: Diode switching losses are included in the IGBT losses with the datasheets I've been using
  note: CHECK FOR IO VS IORMS!!!!!
  "V_s (RMS) " : Inport
  V_batt : Inport  Port=2
  PF : Inport  Port=3
  Idemand (RMS) : Inport  Port=4
  Temp (Ra) : Inport  Port=5
  T_ref (lbs-ft) pass-through : Inport  Port=6
  S_mech (Pass-through) : Inport  Port=7
  Catatrophic Fault Toggle : Inport  Port=8
  Catastrophic Fault Block{1..8} (8 alike) : $bdroot/Catastrophic Fault Block  SystemSampleTime=-1  VariantActivationTime=update diagram  Latency=0  AutoFrameSizeCalculation=off
  Diode Conduction Losses : Subsystem
  Diode Switching Losses : Subsystem  Commented=through
  Display1 : Display
  Divide : Product  Inputs=*/
  Divide1 : Product  Inputs=*/
  Gain : Gain  Gain=6
  Gain1 : Gain  Gain=1/pi
  IGBT Conduction Losses : Subsystem
  IGBT Switching Losses : Subsystem
  I_Ripple : Subsystem
  P_in_mot : Subsystem
  RMS to Max : Gain  Gain=sqrt(2)
  Rankine to Celsius : $bdroot/Rankine to Celsius  SystemSampleTime=-1  VariantActivationTime=update diagram  Latency=0  AutoFrameSizeCalculation=off
  Sum : Sum  Inputs=+++
  Sum1 : Sum
  Sum2 : Sum  Inputs=-+
  Voltage Catastrophic Fault Block : $bdroot/Voltage Catastrophic Fault Block  SystemSampleTime=-1  VariantActivationTime=update diagram  Latency=0  AutoFrameSizeCalculation=off
  mVal : Subsystem
  P_demanded_PWM (W) : Outport  VectorParamsAs1DForOutWhenUnconnected=off
  P_demanded (W) : Outport  Port=2  VectorParamsAs1DForOutWhenUnconnected=off
  Idemanded : Outport  Port=3  VectorParamsAs1DForOutWhenUnconnected=off
  I_Rip : Outport  Port=4  VectorParamsAs1DForOutWhenUnconnected=off
  T_ref (lbs-ft) passed : Outport  Port=5  VectorParamsAs1DForOutWhenUnconnected=off
  S_mech_passed : Outport  Port=6  VectorParamsAs1DForOutWhenUnconnected=off
  V_batt_passed : Outport  Port=7  VectorParamsAs1DForOutWhenUnconnected=off
  eff : Outport  Port=8  VectorParamsAs1DForOutWhenUnconnected=off
  wires:
  Idemand (RMS)/1 -> P_in_mot/2(I), RMS to Max/1
  RMS to Max/1 -> Gain1/1, Diode Conduction Losses/1(I_M), IGBT Conduction Losses/1(I_M)  "I_o"
  IGBT Conduction Losses/1(P_CT) -> Sum/1
  Sum/1 -> Gain/1
  Gain/1 -> Sum1/1, Catastrophic Fault Block8/2, Sum2/1
  PF/1 -> P_in_mot/3(PF), Diode Conduction Losses/2(PF), IGBT Conduction Losses/2(PF)
  mVal/1(m) -> Diode Conduction Losses/3(m), IGBT Conduction Losses/3(m)
  P_in_mot/1(P_in_mot) -> Sum1/2
  Gain1/1 -> IGBT Switching Losses/1(I_ce)
  IGBT Switching Losses/1(P_ST) -> Sum/3
  Diode Conduction Losses/1(P_CD) -> Sum/2
  Temp (Ra)/1 -> Rankine to Celsius/1
  Sum1/1 -> Divide/1, Catastrophic Fault Block2/2, Sum2/2, Divide1/2
  Sum2/1 -> Divide1/1
  Rankine to Celsius/1 -> IGBT Switching Losses/2(T), Diode Conduction Losses/4(T), IGBT Conduction Losses/4(T)
  [FT] -> Catastrophic Fault Block8/1
  Catastrophic Fault Block8/1 -> P_demanded_PWM (W)/1
  [FT] -> Catastrophic Fault Block1/1
  Divide1/1 -> Catastrophic Fault Block1/2
  Catastrophic Fault Block1/1 -> eff/1
  [FT] -> Catastrophic Fault Block2/1
  Catastrophic Fault Block2/1 -> P_demanded (W)/1
  [FT] -> Catastrophic Fault Block3/1
  Divide/1 -> Catastrophic Fault Block3/2
  Catastrophic Fault Block3/1 -> Idemanded/1
  [FT] -> Catastrophic Fault Block4/1
  I_Ripple/1(Inport Value) -> Catastrophic Fault Block4/2  "I_Rip"
  Catastrophic Fault Block4/1 -> I_Rip/1
  "V_s (RMS) "/1 -> mVal/1(V_s), P_in_mot/1(V_s), I_Ripple/2("V_M ")
  Catastrophic Fault Block5/1 -> V_batt_passed/1
  [FT] -> Catastrophic Fault Block5/1
  mVal/2(V_batt_pass) -> Catastrophic Fault Block5/2, Display1/1
  Voltage Catastrophic Fault Block/2 -> mVal/2(V_batt), I_Ripple/1(V_batt), Divide/2
  V_batt/1 -> Voltage Catastrophic Fault Block/2
  Catatrophic Fault Toggle/1 -> Voltage Catastrophic Fault Block/1
  Voltage Catastrophic Fault Block/1 -> [FT]
  T_ref (lbs-ft) pass-through/1 -> Catastrophic Fault Block6/2
  Catastrophic Fault Block6/1 -> T_ref (lbs-ft) passed/1
  [FT] -> Catastrophic Fault Block6/1
  [FT] -> Catastrophic Fault Block7/1
  S_mech (Pass-through)/1 -> Catastrophic Fault Block7/2
  Catastrophic Fault Block7/1 -> S_mech_passed/1

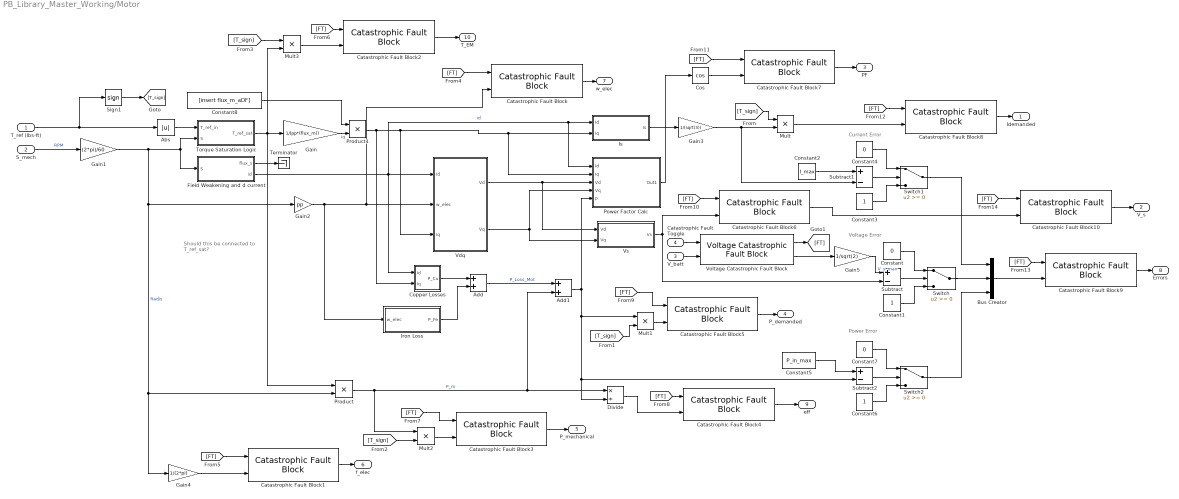
== system PB_Library_Master_Working/Motor ==
  note: Voltage Error
  note: Current Error
  note: Should this be connected
      | to T_ref_sat?
  note: Power Error
  T_ref (lbs-ft) : Inport
  S_mech : Inport  Port=2
  V_batt : Inport  Port=3
  Catastrophic Fault Toggle : Inport  Port=4
  Abs : Abs
  Add : Sum
  Add1 : Sum
  Bus Creator : BusCreator  Inputs=3
  Catastrophic Fault Block{,1..10} (11 alike) : $bdroot/Catastrophic Fault Block  SystemSampleTime=-1  VariantActivationTime=update diagram  Latency=0  AutoFrameSizeCalculation=off
  Constant : Constant  Value=0
  Constant1 : Constant
  Constant2 : Constant  Value=I_max
  Constant3 : Constant
  Constant4 : Constant  Value=0
  Constant5 : Constant  Value=P_in_max
  Constant6 : Constant
  Constant7 : Constant  Value=0
  Constant8 : Constant  Value=[insert flux_m_aDF]
  Copper Losses : Subsystem
  Cos : Trigonometry  Operator=cos
  Divide : Product  Inputs=*/
  "Field Weakening and d current " : Subsystem
  Gain : Gain  Gain=1/(pp*(flux_m))
  Gain1 : Gain  Gain=(2*pi)/60
  Gain2 : Gain  Gain=pp
  Gain3 : Gain  Gain=1/(sqrt(3))
  Gain4 : Gain  Gain=1/(2*pi)
  Gain5 : Gain  Gain=1/sqrt(2)
  Iron Loss : Subsystem
  Is : Subsystem
  Mult{,1..3} (4 alike) : Product  Inputs=**
  "Power Factor Calc " : Subsystem
  Product : Product
  Product1 : Product
  Sign1 : Signum
  Subtract : Sum  Inputs=+-
  Subtract1 : Sum  Inputs=+-
  Subtract2 : Sum  Inputs=+-
  Switch : Switch
  Switch1 : Switch
  Switch2 : Switch
  Terminator : Terminator
  Torque Saturation Logic : Subsystem
  Vdq : Subsystem
  Voltage Catastrophic Fault Block : $bdroot/Voltage Catastrophic Fault Block  SystemSampleTime=-1  VariantActivationTime=update diagram  Latency=0  AutoFrameSizeCalculation=off
  Vs : Subsystem
  Idemanded : Outport  VectorParamsAs1DForOutWhenUnconnected=off
  V_s : Outport  Port=2  VectorParamsAs1DForOutWhenUnconnected=off
  PF : Outport  Port=3  VectorParamsAs1DForOutWhenUnconnected=off
  P_demanded : Outport  Port=4  VectorParamsAs1DForOutWhenUnconnected=off
  P_mechanical : Outport  Port=5  VectorParamsAs1DForOutWhenUnconnected=off
  f_elec : Outport  Port=6  VectorParamsAs1DForOutWhenUnconnected=off
  w_elec : Outport  Port=7  VectorParamsAs1DForOutWhenUnconnected=off
  Errors : Outport  Port=8  VectorParamsAs1DForOutWhenUnconnected=off
  eff : Outport  Port=9  VectorParamsAs1DForOutWhenUnconnected=off
  T_EM : Outport  Port=10  VectorParamsAs1DForOutWhenUnconnected=off
  wires:
  [T_sign] -> Mult3/1
  [T_sign] -> Mult2/2
  [T_sign] -> Mult1/2
  Abs/1 -> Torque Saturation Logic/1(T_ref_in)
  Add/1 -> Add1/1  "P_Loss_Mot"
  Add1/1 -> Divide/2, Subtract2/2, Mult1/1, "Power Factor Calc "/5(P)
  [T_sign] -> Mult/1
  Sign1/1 -> [T_sign]
  "Field Weakening and d current "/2(id) -> "Power Factor Calc "/1(Id), Is/1(Id), Vdq/1(Id), Copper Losses/1(Id)  "id"
  Gain3/1 -> Mult/2, Subtract1/2
  Gain2/1 -> Catastrophic Fault Block/2, Vdq/2(w_elec), Iron Loss/1(w_elec)
  Torque Saturation Logic/1(T_ref_sat) -> Gain/1, Product/1, Mult3/2
  Gain1/1 -> Product/2, Gain4/1, Gain2/1, "Field Weakening and d current "/1(S), Torque Saturation Logic/2(S)  "Rad/s"
  Copper Losses/1(P_Cu) -> Add/1
  Iron Loss/1(P_Fe) -> Add/2
  Product/1 -> Divide/1, Add1/2, Mult2/1  "P_m"
  Vdq/1(Vd) -> "Power Factor Calc "/3(Vd), Vs/1(Vd)
  Vdq/2(Vq) -> "Power Factor Calc "/4(Vq), Vs/2(Vq)
  Is/1(Is) -> Gain3/1
  Vs/1(Vs) -> Subtract/2, Catastrophic Fault Block6/2
  "Power Factor Calc "/1(Out1) -> Cos/1
  Gain5/1 -> Subtract/1  "V_s_max"
  Subtract/1 -> Switch/2
  Constant/1 -> Switch/1
  Constant1/1 -> Switch/3
  Switch/1 -> Bus Creator/2
  Constant2/1 -> Subtract1/1
  Switch1/1 -> Bus Creator/1
  Constant3/1 -> Switch1/3
  Constant4/1 -> Switch1/1
  Subtract1/1 -> Switch1/2
  Constant7/1 -> Switch2/1
  Constant5/1 -> Subtract2/1
  Subtract2/1 -> Switch2/2
  Constant6/1 -> Switch2/3
  Switch2/1 -> Bus Creator/3
  Catastrophic Fault Block/1 -> w_elec/1
  [FT] -> Catastrophic Fault Block/1
  [FT] -> Catastrophic Fault Block1/1
  Gain4/1 -> Catastrophic Fault Block1/2
  Catastrophic Fault Block1/1 -> f_elec/1
  [FT] -> Catastrophic Fault Block2/1
  Mult3/1 -> Catastrophic Fault Block2/2
  Catastrophic Fault Block2/1 -> T_EM/1
  [FT] -> Catastrophic Fault Block3/1
  Mult2/1 -> Catastrophic Fault Block3/2
  Catastrophic Fault Block3/1 -> P_mechanical/1
  [FT] -> Catastrophic Fault Block4/1
  Divide/1 -> Catastrophic Fault Block4/2
  Catastrophic Fault Block4/1 -> eff/1
  [FT] -> Catastrophic Fault Block5/1
  Mult1/1 -> Catastrophic Fault Block5/2
  Catastrophic Fault Block5/1 -> P_demanded/1
  [FT] -> Catastrophic Fault Block6/1
  [FT] -> Catastrophic Fault Block7/1
  Cos/1 -> Catastrophic Fault Block7/2
  Catastrophic Fault Block7/1 -> PF/1
  [FT] -> Catastrophic Fault Block8/1
  Mult/1 -> Catastrophic Fault Block8/2
  Catastrophic Fault Block8/1 -> Idemanded/1
  [FT] -> Catastrophic Fault Block9/1
  Bus Creator/1 -> Catastrophic Fault Block9/2
  Catastrophic Fault Block9/1 -> Errors/1
  [FT] -> Catastrophic Fault Block10/1
  Catastrophic Fault Block6/1 -> Catastrophic Fault Block10/2
  Catastrophic Fault Block10/1 -> V_s/1
  "Field Weakening and d current "/1(flux_s) -> Terminator/1
  Gain/1 -> Product1/2  "iq"
  Product1/1 -> Copper Losses/2(Iq), Vdq/3(Iq), "Power Factor Calc "/2(Iq), Is/2(Iq)
  Constant8/1 -> Product1/1
  T_ref (lbs-ft)/1 -> Sign1/1, Abs/1
  S_mech/1 -> Gain1/1  "RPM"
  Voltage Catastrophic Fault Block/2 -> Gain5/1
  Catastrophic Fault Toggle/1 -> Voltage Catastrophic Fault Block/1
  Voltage Catastrophic Fault Block/1 -> [FT]
  V_batt/1 -> Voltage Catastrophic Fault Block/2

== system PB_Library_Master_Working/Rankine to Celsius ==
  Rankine : Inport
  Add : Sum  Inputs=+-
  Constant : Constant  Value=491.67
  Constant1 : Constant  Value=1.8
  Divide : Product  Inputs=*/
  Celsius : Outport
  wires:
  Divide/1 -> Celsius/1
  Rankine/1 -> Add/1
  Constant/1 -> Add/2
  Add/1 -> Divide/1
  Constant1/1 -> Divide/2

== system PB_Library_Master_Working/Rectifier ==
  note: -------------------------------------------------------
      | Created by Nathan Butler and Mark Bell
      | NASA Glenn Research Center
      | MATLAB R2020b
      | Spring 2021
      |
      | Design derived from EMTAT PB Inverter
      | -------------------------------------------------------
  Idemand : Inport
  "V_s (RMS) " : Inport  Port=2
  PF : Inport  Port=3
  Temp (Ra) : Inport  Port=4
  V_batt (Standin) : Inport  Port=5
  Catastrophic Fault Toggle : Inport  Port=6
  Catastrophic Fault Block{,1..5} (6 alike) : $bdroot/Catastrophic Fault Block  SystemSampleTime=-1  VariantActivationTime=update diagram  Latency=0  AutoFrameSizeCalculation=off
  Diode Conduction Losses1 : Subsystem
  Divide2 : Product  Inputs=*/
  Divide3 : Product  Inputs=*/
  Gain2 : Gain  Gain=6
  Gain3 : Gain  Gain=1/pi
  IGBT Conduction Losses1 : Subsystem
  IGBT Switching Losses1 : Subsystem
  I_Ripple1 : Subsystem
  Math : Gain  Gain=1/sqrt(2)
  P_out_gen : Subsystem
  "RMS to V_batt " : Gain  Gain=sqrt(2)
  Rankine to Celsius : $bdroot/Rankine to Celsius  SystemSampleTime=-1  VariantActivationTime=update diagram  Latency=0  AutoFrameSizeCalculation=off
  Sum3 : Sum
  Sum4 : Sum  Inputs=+++
  Sum5 : Sum  Inputs=-+
  Terminator : Terminator
  Voltage Catastrophic Fault Block : $bdroot/Voltage Catastrophic Fault Block  SystemSampleTime=-1  VariantActivationTime=update diagram  Latency=0  AutoFrameSizeCalculation=off
  mVal : Subsystem
  to I_RMS : Gain  Gain=1/sqrt(2)
  P_demanded_PWM (W) : Outport  VectorParamsAs1DForOutWhenUnconnected=off
  P_demanded (W) : Outport  Port=2  VectorParamsAs1DForOutWhenUnconnected=off
  Idemanded (RMS) : Outport  Port=3  VectorParamsAs1DForOutWhenUnconnected=off
  I_Rip : Outport  Port=4  VectorParamsAs1DForOutWhenUnconnected=off
  V_out : Outport  Port=5  VectorParamsAs1DForOutWhenUnconnected=off
  eff : Outport  Port=6  VectorParamsAs1DForOutWhenUnconnected=off
  wires:
  Rankine to Celsius/1 -> IGBT Conduction Losses1/4(T), IGBT Switching Losses1/2(T), Diode Conduction Losses1/4(T)
  "RMS to V_batt "/1 -> Catastrophic Fault Block4/2, Divide2/2, I_Ripple1/1(V_batt), mVal/2(V_batt)  "V_batt"
  Divide2/1 -> Math/1  "Idemanded"
  P_out_gen/1(P_out_gen) -> Sum3/1  "P_out_gen"
  Gain2/1 -> Sum3/2, Catastrophic Fault Block/2, Sum5/1  "P_demanded_PWM"
  Idemand/1 -> IGBT Conduction Losses1/1(I_M), Gain3/1, Diode Conduction Losses1/1(I_M), to I_RMS/1  "Idemand"
  PF/1 -> P_out_gen/3(PF), Diode Conduction Losses1/2(PF), IGBT Conduction Losses1/2(PF)  "PF"
  mVal/1(m) -> Diode Conduction Losses1/3(m), IGBT Conduction Losses1/3(m)  "(=1)"
  Diode Conduction Losses1/1(P_CD) -> Sum4/2
  Sum4/1 -> Gain2/1
  IGBT Conduction Losses1/1(P_CT) -> Sum4/1
  IGBT Switching Losses1/1(P_ST) -> Sum4/3
  Gain3/1 -> IGBT Switching Losses1/1(I_ce)
  Temp (Ra)/1 -> Rankine to Celsius/1  "Temp (Ra)"
  Sum3/1 -> Catastrophic Fault Block2/2, Divide3/2, Sum5/2, Divide2/1  "P_demanded"
  Sum5/1 -> Divide3/1
  to I_RMS/1 -> P_out_gen/1(I (RMS))
  V_batt (Standin)/1 -> Terminator/1  "V_batt"
  Catastrophic Fault Block/1 -> P_demanded_PWM (W)/1
  [FT] -> Catastrophic Fault Block/1
  [FT] -> Catastrophic Fault Block1/1
  Divide3/1 -> Catastrophic Fault Block1/2  "eff"
  Catastrophic Fault Block1/1 -> eff/1
  [FT] -> Catastrophic Fault Block2/1
  Catastrophic Fault Block2/1 -> P_demanded (W)/1
  [FT] -> Catastrophic Fault Block3/1
  Math/1 -> Catastrophic Fault Block3/2
  Catastrophic Fault Block3/1 -> Idemanded (RMS)/1
  [FT] -> Catastrophic Fault Block4/1
  Catastrophic Fault Block4/1 -> V_out/1
  [FT] -> Catastrophic Fault Block5/1
  I_Ripple1/1(I_Rip) -> Catastrophic Fault Block5/2  "I_Rip"
  Catastrophic Fault Block5/1 -> I_Rip/1
  Voltage Catastrophic Fault Block/2 -> "RMS to V_batt "/1, I_Ripple1/2("V_M "), mVal/1(V_s), P_out_gen/2(V_s (RMS))
  Voltage Catastrophic Fault Block/1 -> [FT]
  Catastrophic Fault Toggle/1 -> Voltage Catastrophic Fault Block/1
  "V_s (RMS) "/1 -> Voltage Catastrophic Fault Block/2  "V_s (RMS)"

== system PB_Library_Master_Working/Resistor_I ==
  Idemand : Inport
  Resistance : Inport  Port=2
  Temp (Rankine) : Inport  Port=3  Unit=degC
  FaultToggle : Inport  Port=4  Unit=degC
  Catastrophic Fault Block : $bdroot/Catastrophic Fault Block  SystemSampleTime=-1  VariantActivationTime=update diagram  Latency=0  AutoFrameSizeCalculation=off
  Catastrophic Fault Block1 : $bdroot/Catastrophic Fault Block  SystemSampleTime=-1  VariantActivationTime=update diagram  Latency=0  AutoFrameSizeCalculation=off
  Catastrophic Fault Block2 : $bdroot/Catastrophic Fault Block  SystemSampleTime=-1  VariantActivationTime=update diagram  Latency=0  AutoFrameSizeCalculation=off
  Constant : Constant  Value=[insert resistance_aDF]
  Multiply : Product
  Multiply1 : Product
  Product1 : Product
  Rankine to Celsius : $bdroot/Rankine to Celsius  SystemSampleTime=-1  VariantActivationTime=update diagram  Latency=0  AutoFrameSizeCalculation=off
  Terminator : Terminator
  VDrop : Outport  VectorParamsAs1DForOutWhenUnconnected=off
  Idemanded : Outport  Port=2  VectorParamsAs1DForOutWhenUnconnected=off
  Heat : Outport  Port=3  VectorParamsAs1DForOutWhenUnconnected=off
  wires:
  Multiply/1 -> Multiply1/1, Catastrophic Fault Block/2
  Temp (Rankine)/1 -> Rankine to Celsius/1
  Rankine to Celsius/1 -> Terminator/1
  FaultToggle/1 -> [FT]
  [FT] -> Catastrophic Fault Block/1
  Catastrophic Fault Block/1 -> VDrop/1
  [FT] -> Catastrophic Fault Block1/1
  Catastrophic Fault Block1/1 -> Idemanded/1
  [FT] -> Catastrophic Fault Block2/1
  Multiply1/1 -> Catastrophic Fault Block2/2
  Catastrophic Fault Block2/1 -> Heat/1
  Idemand/1 -> Multiply1/2, Catastrophic Fault Block1/2, Multiply/2
  Constant/1 -> Product1/1
  Resistance/1 -> Product1/2
  Product1/1 -> Multiply/1

== system PB_Library_Master_Working/Resistor_V ==
  "VDrop " : Inport
  "Resistance " : Inport  Port=2
  Temp : Inport  Port=3  Unit=degC
  FaultToggle : Inport  Port=4  Unit=degC
  Catastrophic Fault Block : $bdroot/Catastrophic Fault Block  SystemSampleTime=-1  VariantActivationTime=update diagram  Latency=0  AutoFrameSizeCalculation=off
  Catastrophic Fault Block1 : $bdroot/Catastrophic Fault Block  SystemSampleTime=-1  VariantActivationTime=update diagram  Latency=0  AutoFrameSizeCalculation=off
  Constant : Constant  Value=[insert resistance_aDF]
  Divide : Product  Inputs=*/
  Multiply1 : Product
  Product : Product
  Rankine to Celsius : $bdroot/Rankine to Celsius  SystemSampleTime=-1  VariantActivationTime=update diagram  Latency=0  AutoFrameSizeCalculation=off
  Terminator : Terminator
  Idemand : Outport  VectorParamsAs1DForOutWhenUnconnected=off
  Heat : Outport  Port=2  VectorParamsAs1DForOutWhenUnconnected=off
  wires:
  "VDrop "/1 -> Multiply1/1, Divide/1
  Divide/1 -> Catastrophic Fault Block/2, Multiply1/2
  Temp/1 -> Rankine to Celsius/1
  Rankine to Celsius/1 -> Terminator/1
  FaultToggle/1 -> [FT]
  [FT] -> Catastrophic Fault Block/1
  Catastrophic Fault Block/1 -> Idemand/1
  Multiply1/1 -> Catastrophic Fault Block1/2
  [FT] -> Catastrophic Fault Block1/1
  Catastrophic Fault Block1/1 -> Heat/1
  Product/1 -> Divide/2
  "Resistance "/1 -> Product/2
  Constant/1 -> Product/1

== system PB_Library_Master_Working/Voltage Catastrophic Fault Block ==
  Inport Fault Toggle : Inport
  Inport Voltage : Inport  Port=2
  Display{,1..3} (4 alike) : Display
  IsNonZero : simulink/Logic and Bit Operations/Compare To Zero  relop=~=  OutDataTypeStr=boolean
  IsZero : simulink/Logic and Bit Operations/Compare To Zero  relop===  OutDataTypeStr=boolean
  IsZero1 : simulink/Logic and Bit Operations/Compare To Zero  relop===  OutDataTypeStr=boolean
  OR : Logic  Operator=OR  IconShape=distinctive  AllPortsSameDT=off  OutDataTypeStr=boolean
  Switch : Switch  Criteria=u2 > Threshold
  Switch1 : Switch  Criteria=u2 > Threshold
  Zero1 : Constant
  Zero2 : Constant  Value=0
  Outport Fault Toggle : Outport
  Outport Voltage : Outport  Port=2
  wires:
  Switch1/1 -> Outport Voltage/1, Display3/1, IsZero1/1
  Inport Voltage/1 -> IsZero/1, Switch1/3
  Zero2/1 -> Switch1/1
  IsZero1/1 -> Switch/2
  Switch/1 -> Outport Fault Toggle/1, Display1/1
  [FT] -> Switch/3
  Zero1/1 -> Switch/1
  IsZero/1 -> Display2/1, OR/2
  IsNonZero/1 -> OR/1, Display/1
  OR/1 -> Switch1/2
  Inport Fault Toggle/1 -> [FT]
  [FT] -> IsNonZero/1

== system PB_Library_Master_Working/Boost Converter/DC - DC Converter ==
  note: Power B
  note: Current B
  note: Power A
  NodeA : Inport
  IAg : Inport  Port=2
  x : Inport  Port=3
  d : Inport  Port=4
  dt : Inport  Port=5
  Iout : Inport  Port=6
  P loss : Inport  Port=7
  "T_Ambient " : Inport  Port=8
  " Dynamic State" : Subsystem  TreatAsAtomicUnit=on
  "1=dynamic, 0=static" : Display
  Add : Sum  Inputs=+-
  Bus Creator1 : BusCreator  Inputs=3
  Bus Creator3 : BusCreator  Inputs=3
  Bus Selector : BusSelector  OutputSignals=x,xdot,VB
  Constant : Constant  Value=[0, 1/C_M; -1/L_M, -(Ron_M+RC_M+RL_M)/L_M]  VectorParams1D=off
  Display : Display
  Divide : Product  Commented=on  Inputs=*/
  Goto12 : Goto  Commented=on  GotoTag=IB
  Goto14 : From  Commented=on  GotoTag=PwrB
  Goto15 : From  Commented=on  GotoTag=VB
  Goto5 : From  Commented=on  GotoTag=IB
  If : If
  MATLAB Function : MATLAB Function  TreatAsAtomicUnit=on
  Mux : Mux  Inputs=2
  Negate : Gain  Commented=through  Gain=-1
  Product3 : Product
  Steady State : Subsystem  TreatAsAtomicUnit=on
  Switch : Switch  Criteria=u2 ~= 0
  xdot : Constant  Value=zeros(2,1)  VectorParams1D=off
  NodeB : Outport  VectorParamsAs1DForOutWhenUnconnected=off
  x_dot : Outport  Port=2  VectorParamsAs1DForOutWhenUnconnected=off
  x_new : Outport  Port=3  VectorParamsAs1DForOutWhenUnconnected=off
  PElec : Outport  Port=4  VectorParamsAs1DForOutWhenUnconnected=off
  IA : Outport  Port=5  VectorParamsAs1DForOutWhenUnconnected=off
  switchDyn : Outport  Port=6  VectorParamsAs1DForOutWhenUnconnected=off
  wires:
  [PwrB] -> PElec/1
  "T_Ambient "/1 -> Steady State/3("T_Ambient "), Display/1
  Negate/1 -> [PwrB]
  Mux/1 -> " Dynamic State"/2(u), Steady State/1(u)
  Iout/1 -> Mux/2
  [VA] -> Mux/1
  [x] -> x_new/1
  Bus Creator3/1 -> Switch/1
  Bus Selector/1 -> [x]  "<x>"
  Bus Selector/2 -> [xdot]  "<xdot>"
  Bus Selector/3 -> [VB]  "<VB>"
  xdot/1 -> Bus Creator1/2  "xdot"
  Steady State/2(VB) -> Bus Creator1/3  "VB"
  " Dynamic State"/1(xdot) -> Bus Creator3/2  "xdot"
  " Dynamic State"/2(VB) -> Bus Creator3/3  "VB"
  Switch/1 -> Bus Selector/1
  Add/1 -> Negate/1
  P loss/1 -> Add/2
  [PwrA] -> Add/1
  [xdot] -> x_dot/1
  d/1 -> " Dynamic State"/3(d), Steady State/2(d)
  x/1 -> " Dynamic State"/1(x), Bus Creator3/1  "x"
  Steady State/1(x) -> Bus Creator1/1  "x"
  dt/1 -> MATLAB Function/2(dt)
  If/2 -> Steady State/Action
  Constant/1 -> MATLAB Function/1(A1)
  If/1 -> " Dynamic State"/Action
  MATLAB Function/1(y) -> If/1, switchDyn/1, Switch/2, "1=dynamic, 0=static"/1
  [IA] -> IA/1
  Goto5/1 -> ?  "I"
  IAg/1 -> [IA]
  Goto15/1 -> Divide/2
  Divide/1 -> Goto12/1
  Goto14/1 -> Divide/1
  [IA] -> Product3/2
  NodeA/1 -> [VA]
  [VB] -> NodeB/1  "V"
  Product3/1 -> [PwrA]
  [VA] -> Product3/1
  Bus Creator1/1 -> Switch/3
